simulink model "dynamics_point"  (R2021b)
settings: Solver=VariableStepAuto  StartTime=0.0  StopTime=60  RelTol=1e-10  AbsTol=1e-14
values from neighbouring files (symbols this model uses):
  q0 = [-0.8;0;pi]    [SIM01.m]    (also in SIM02.m = [j 0 the(k)]'; SIM03.m = [-1;0;-pi/2]; SIM04.m = [1 1 k]'; SIM05.m = [2;1;2])
  s0 = [0;0]    [SIM01.m]    (also in SIM02.m; SIM06.m)
  V0 = [0;0]    [SIM06.m]    (also in SIM07.m)
settings Model: Creator=PC  LastModifiedBy=PC
settings DataIOCC: SaveFormat=Array

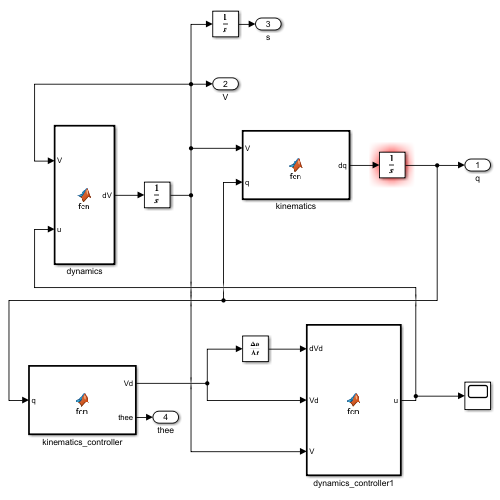
[thumbnail: Simulink's stored preview of the top-level diagram]
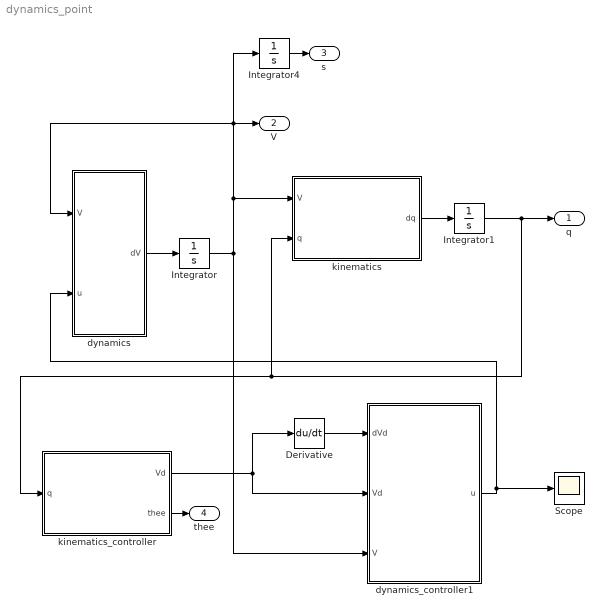
== system dynamics_point ==
  Derivative : Derivative
  Integrator : Integrator  InitialCondition=V0
  Integrator1 : Integrator  InitialCondition=q0
  Integrator4 : Integrator  InitialCondition=s0
  Scope : Scope
  dynamics : MATLAB Function  TreatAsAtomicUnit=on
  dynamics_controller1 : MATLAB Function  TreatAsAtomicUnit=on
  kinematics : MATLAB Function  TreatAsAtomicUnit=on
  kinematics_controller : MATLAB Function  TreatAsAtomicUnit=on
  q : Outport
  V : Outport  Port=2
  s : Outport  Port=3
  thee : Outport  Port=4
  wires:
  dynamics/1(dV) -> Integrator/1
  Integrator/1 -> dynamics_controller1/3(V), kinematics/1(V), Integrator4/1, V/1, dynamics/1(V)
  kinematics_controller/1(Vd) -> dynamics_controller1/2(Vd), Derivative/1
  Derivative/1 -> dynamics_controller1/1(dVd)
  Integrator1/1 -> q/1, kinematics/2(q), kinematics_controller/1(q)
  dynamics_controller1/1(u) -> Scope/1, dynamics/2(u)
  kinematics_controller/2(thee) -> thee/1
  Integrator4/1 -> s/1
  kinematics/1(dq) -> Integrator1/1

== matlab function dynamics_point/dynamics ==
  data: V input size=2*1; u input size=2*1; dV output size=2*1
function dV = fcn(V,u)
m=3;
p=0.1;
J=1;
d=0.05;
r=0.05;
L=0.1;
al=m+p;
be=m*d^2+p*L^2+J;
ga=m*d;
M=diag([al,be]);
dV = M^-1*(ga*V(2)*[V(2);-V(1)]+[1 1;L -L]*u/r);

== matlab function dynamics_point/kinematics ==
  data: V input size=2*1; dq output size=3*1; q input size=3*1
function dq = fcn(V,q)
dq=[ cos(q(3))  0
     sin(q(3))  0
      0         1]*V;

== matlab function dynamics_point/kinematics_controller ==
  data: q input size=3*1; Vd output size=2*1; thee output size=1
function [Vd,thee]= fcn(q)

the=atan2(sin(q(3)),cos(q(3)));

k1=0.2;k2=0.375;
vm=0.05;wm=0.78;

al=atan2(-q(2),-q(1));    
thee=atan2(sin(al-the),cos(al-the));
d=sqrt(q(2)^2+q(1)^2);
vp=k1*d;
vd=vp*cos(thee*0.5)^2;
v=min(vd,vm);
dal=v*sin(thee)/d;
wd=dal+2*k2*sin(thee*0.5);
w=sign(wd)*min(abs(wd),wm);
Vd=[v;w];

== matlab function dynamics_point/dynamics_controller1 ==
  data: dVd input size=2*1; u output size=2*1; Vd input size=2*1; V input size=2*1
function u= fcn(dVd,Vd,V)
K=5;
m=3;
p=0.1;
J=1;
d=0.05;
r=0.05;
L=0.1;
al=m+p;
be=m*d^2+p*L^2+J;
ga=m*d;
M=diag([al,be]);
dV=dVd-K*(V-Vd);
C=[1 1;L -L]/r;
u=C^-1*(M*dV-ga*V(2)*[V(2);-V(1)]);
